simulink model "PolePlacement"  (R2023a)
settings: Solver=VariableStepAuto  StartTime=0.0  StopTime=10.0  RelTol=1e-3
settings Model: Creator=bl4ck  LastModifiedBy=bl4ck

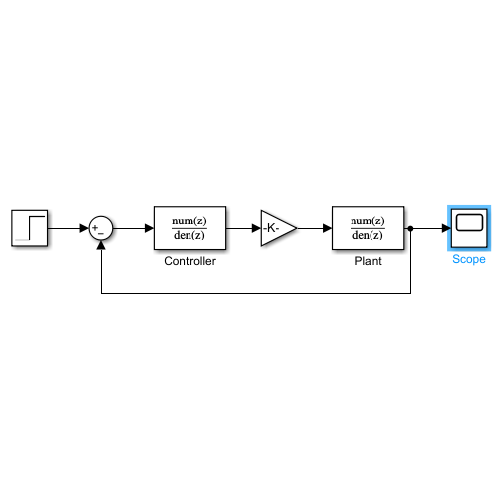
[thumbnail: Simulink's stored preview of the top-level diagram]
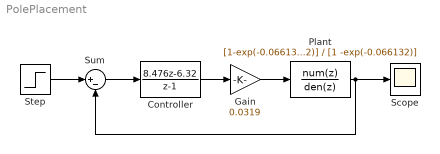
== system PolePlacement ==
  Controller : DiscreteTransferFcn  Numerator=[8.476 -6.32]  Denominator=[1 -1]  SampleTime=0.01
  Gain : Gain  Gain=0.0319
  Plant : DiscreteTransferFcn  Numerator=[1-exp(-0.066132)]  Denominator=[1 -exp(-0.066132)]  SampleTime=0.01
  Scope : Scope
  Step : Step  After=10  SampleTime=0
  Sum : Sum  Inputs=|+-
  wires:
  Step/1 -> Sum/1
  Sum/1 -> Controller/1
  Controller/1 -> Gain/1
  Gain/1 -> Plant/1
  Plant/1 -> Sum/2, Scope/1
